simulink library "IAM_Table"  (Simulink 8.2)
settings: Solver=ode45  StartTime=0.0  StopTime=10.0  RelTol=1e-3
settings Model: Creator=lena.frank  LastModifiedBy=drhf

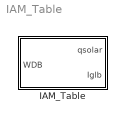
== system IAM_Table ==
  IAM_Table : Subsystem  mask(IAM Table for Solar Thermal Collectors){fta=0.8, angle=[0:5:90], Kb=[1.0000    1.0000    0.9999    0.9996    0.9991    0.9982    0.9965  0.9935    0.9886    0.9807    0.9678    0.9473    0.9148    0.8638   0.7846    0.6644    0.4907    0.2599    0.0000], Kd=0.92}
      mask prompts: fta "Fin Efficiency * Transmission * Absorption (FTA) [-]"; angle "Direct incidence angles for IAM [degree]"; Kb "Kdir: Incidence angle modifier direct radiation (0..1)"; Kd "Kdfu : Incidence angle modifier diffuse radiation"
      mask help:
      | Transforms direct and diffuse radiation to an absorbed solar power per unit area. The direct radiation incidence angle modifier (Kdir) uses the table-model for collectors (EN 12975).
      | FTA or F'(TauAlfa) is defined from the incidence angle modifiers Kdir and Kdfu:
      | FTA = eta0 / (Kdir(15°)*0.85 + Kdfu*0.15)
      | Direct radiation: Kdir and the incidence angle are vectors
      | Diffuse radiation  Kdfu = constant (at 50° incidence)
      mask Help: web(fullfile(path_carnot('help'),'IAM_Table.html'),'-helpbrowser')

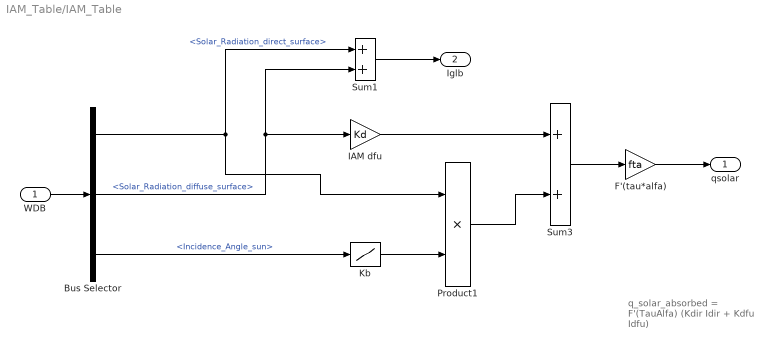
== system IAM_Table/IAM_Table ==
  note: q_solar_absorbed = F'(TauAlfa) (Kdir Idir + Kdfu Idfu)
  WDB : Inport
  Bus Selector : BusSelector  OutputSignals=Solar_Radiation_direct_surface,Solar_Radiation_diffuse_surface,Incidence_Angle_sun
  F'(tau*alfa) : Gain  Gain=fta  SaturateOnIntegerOverflow=on  OutDataTypeStr=Inherit: Same as input  ParamDataTypeStr=Inherit: Same as input
  IAM dfu : Gain  Gain=Kd  SaturateOnIntegerOverflow=on  OutDataTypeStr=Inherit: Same as input  ParamDataTypeStr=Inherit: Same as input
  Kb : Lookup  InputValues=angle  Table=Kb  SaturateOnIntegerOverflow=on
  Product1 : Product  SaturateOnIntegerOverflow=on  InputSameDT=on  OutDataTypeStr=Inherit: Same as first input
  Sum1 : Sum  SaturateOnIntegerOverflow=on  InputSameDT=on  OutDataTypeStr=Inherit: Same as first input
  Sum3 : Sum  SaturateOnIntegerOverflow=on  InputSameDT=on  OutDataTypeStr=Inherit: Same as first input
  qsolar : Outport
  Iglb : Outport  Port=2
  wires:
  WDB/1 -> Bus Selector/1
  Product1/1 -> Sum3/2
  IAM dfu/1 -> Sum3/1
  Bus Selector/1 -> Sum1/1, Product1/1  "<Solar_Radiation_direct_surface>"
  Bus Selector/2 -> Sum1/2, IAM dfu/1  "<Solar_Radiation_diffuse_surface>"
  Bus Selector/3 -> Kb/1  "<Incidence_Angle_sun>"
  Kb/1 -> Product1/2
  Sum3/1 -> F'(tau*alfa)/1
  Sum1/1 -> Iglb/1
  F'(tau*alfa)/1 -> qsolar/1
